simulink model "mainV02_49"  (R2016b)
settings: Solver=FixedStepAuto  StartTime=0.0  StopTime=inf  FixedStep=Ts  MaxStep=0.2  RelTol=1e-2
undefined symbols (not defined in the file): checks, datetime, decyear, deltae_degrees, deltafl_degrees, deltafr_degrees, deltar_degrees, deltat_1, deltat_2, deltat_3, deltat_4, deltat_5, Earth, F, ft, groundReaction, initialValues, juliandate, LD, leapyear, Light, m, MIL, Newton, Raphson, s, sigbuilder_block, Ts, Vehicle, WGS84
libraries: simulink x25, aerolibutil x17, aerolibtransform2 x12, aerolib6dofsys x5, aerolibasang x4, aerolib6dof2 x4, aerolibwind2 x3, aerolibbdyn x3, aerolibconvert2 x3, aerolibactuator x2, aerolibgravity2 x2, aerolibnav x2
(part 2 of 7)

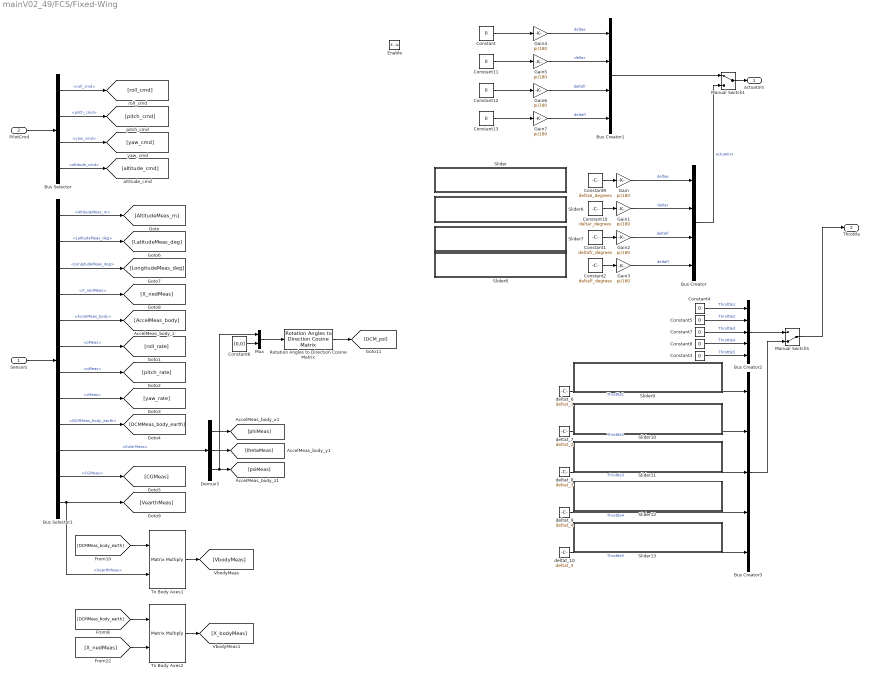
== system mainV02_49/FCS/Fixed-Wing ==
  Sensors : Inport  OutDataTypeStr=Bus: SensorsBus
  PilotCmd : Inport  Port=2  OutDataTypeStr=Bus: CommandBus
  Enable : EnablePort
  Bus Creator : BusCreator  Inputs='deltae','deltar','deltafr','deltafl'  OutDataTypeStr=Bus: ActuatorsBus  NonVirtualBus=on
  Bus Creator1 : BusCreator  Inputs='deltae','deltar','deltafr','deltafl'  OutDataTypeStr=Bus: ActuatorsBus  NonVirtualBus=on
  Bus Creator2 : BusCreator  Inputs='Throttle1','Throttle2','Throttle3','Throttle4','Throttle5'  OutDataTypeStr=Bus: ThrottleBus  NonVirtualBus=on
  Bus Creator3 : BusCreator  Inputs='Throttle1','Throttle2','Throttle3','Throttle4','Throttle5'  OutDataTypeStr=Bus: ThrottleBus  NonVirtualBus=on
  Bus Selector : BusSelector  OutputSignals=roll_cmd,pitch_cmd,yaw_cmd,altitude_cmd
  Bus Selector1 : BusSelector  OutputSignals=LLAMeas.AltitudeMeas_m,LLAMeas.LatitudeMeas_deg,LLAMeas.LongitudeMeas_deg,X_nedMeas,AccelMeas_body,OmegaMeas_body.pMeas,OmegaMeas_body.qMeas,OmegaMeas_body.rMeas,DCMMeas_body_earth,EulerMeas,CGMeas,VearthMeas
  Constant{,3..5,7..8,11..13} (9 alike) : Constant  Value=0
  Constant1 : Constant  Value=deltafr_degrees
  Constant10 : Constant  Value=deltar_degrees
  Constant2 : Constant  Value=deltafl_degrees
  Constant6 : Constant  Value=[0,0]
  Constant9 : Constant  Value=deltae_degrees
  Demux3 : Demux  Outputs=3
  Gain{,1..7} (8 alike) : Gain  Gain=pi/180
  Manual Switch1 : ManualSwitch
  Manual Switch5 : ManualSwitch  CurrentSetting=0
  Mux : Mux  Inputs=2
  Rotation Angles to Direction Cosine Matrix : aerolibtransform2/Rotation Angles to Direction Cosine Matrix  rotationOrder=ZYX
  Slider : Subsystem  DialogController=hmiCreateDDGDialog  IsWebBlock=on  mask(MWDashboardBlock){webBlockId=14b23d13-a400-494b-8ed9-02e5a1d75a92, webBlockType=slider, ShowInLibBrowser=on, ShowInitialText=on, HMISrcModelName=mainV02_49}
      mask prompts: webBlockId "WebBlock Id"; webBlockType "WebBlock Type"; HMISrcModelName "Source Model"
      mask help: SimulinkHMI:dialogs:SliderDialogDesc
      mask Help: helpview([docroot '/mapfiles/simulink.map'], 'hmi_slider')
      mask Display:
      | if strcmp(get_param(bdroot(gcb),'BlockDiagramType'), 'library')
      |     image([(matlabroot) '/toolbox/simulink/hmi/icons/Slider.png']);
      | end
  Slider10 : Subsystem  DialogController=hmiCreateDDGDialog  IsWebBlock=on  mask(MWDashboardBlock){webBlockId=64fa6611-4453-4c5a-8fed-f588a42e496e, webBlockType=slider, ShowInLibBrowser=on, ShowInitialText=on, HMISrcModelName=mainV02_49}
      mask prompts: webBlockId "WebBlock Id"; webBlockType "WebBlock Type"; HMISrcModelName "Source Model"
      mask help: SimulinkHMI:dialogs:SliderDialogDesc
      mask Help: helpview([docroot '/mapfiles/simulink.map'], 'hmi_slider')
      mask Display:
      | if strcmp(get_param(bdroot(gcb),'BlockDiagramType'), 'library')
      |     image([(matlabroot) '/toolbox/simulink/hmi/icons/Slider.png']);
      | end
  Slider11 : Subsystem  DialogController=hmiCreateDDGDialog  IsWebBlock=on  mask(MWDashboardBlock){webBlockId=9533f27f-d213-4a1e-af4f-df3e89cb42b9, webBlockType=slider, ShowInLibBrowser=on, ShowInitialText=on, HMISrcModelName=mainV02_49}
      mask prompts: webBlockId "WebBlock Id"; webBlockType "WebBlock Type"; HMISrcModelName "Source Model"
      mask help: SimulinkHMI:dialogs:SliderDialogDesc
      mask Help: helpview([docroot '/mapfiles/simulink.map'], 'hmi_slider')
      mask Display:
      | if strcmp(get_param(bdroot(gcb),'BlockDiagramType'), 'library')
      |     image([(matlabroot) '/toolbox/simulink/hmi/icons/Slider.png']);
      | end
  Slider12 : Subsystem  DialogController=hmiCreateDDGDialog  IsWebBlock=on  mask(MWDashboardBlock){webBlockId=b1a90b42-9e20-4e98-9400-f4073a2edd03, webBlockType=slider, ShowInLibBrowser=on, ShowInitialText=on, HMISrcModelName=mainV02_49}
      mask prompts: webBlockId "WebBlock Id"; webBlockType "WebBlock Type"; HMISrcModelName "Source Model"
      mask help: SimulinkHMI:dialogs:SliderDialogDesc
      mask Help: helpview([docroot '/mapfiles/simulink.map'], 'hmi_slider')
      mask Display:
      | if strcmp(get_param(bdroot(gcb),'BlockDiagramType'), 'library')
      |     image([(matlabroot) '/toolbox/simulink/hmi/icons/Slider.png']);
      | end
  Slider13 : Subsystem  DialogController=hmiCreateDDGDialog  IsWebBlock=on  mask(MWDashboardBlock){webBlockId=3f53d0a3-a536-4819-a79a-261ce29de858, webBlockType=slider, ShowInLibBrowser=on, ShowInitialText=on, HMISrcModelName=mainV02_49}
      mask prompts: webBlockId "WebBlock Id"; webBlockType "WebBlock Type"; HMISrcModelName "Source Model"
      mask help: SimulinkHMI:dialogs:SliderDialogDesc
      mask Help: helpview([docroot '/mapfiles/simulink.map'], 'hmi_slider')
      mask Display:
      | if strcmp(get_param(bdroot(gcb),'BlockDiagramType'), 'library')
      |     image([(matlabroot) '/toolbox/simulink/hmi/icons/Slider.png']);
      | end
  Slider6 : Subsystem  DialogController=hmiCreateDDGDialog  IsWebBlock=on  mask(MWDashboardBlock){webBlockId=0a8845a4-7a41-4249-8bd0-83b7bb709b45, webBlockType=slider, ShowInLibBrowser=on, ShowInitialText=on, HMISrcModelName=mainV02_49}
      mask prompts: webBlockId "WebBlock Id"; webBlockType "WebBlock Type"; HMISrcModelName "Source Model"
      mask help: SimulinkHMI:dialogs:SliderDialogDesc
      mask Help: helpview([docroot '/mapfiles/simulink.map'], 'hmi_slider')
      mask Display:
      | if strcmp(get_param(bdroot(gcb),'BlockDiagramType'), 'library')
      |     image([(matlabroot) '/toolbox/simulink/hmi/icons/Slider.png']);
      | end
  Slider7 : Subsystem  DialogController=hmiCreateDDGDialog  IsWebBlock=on  mask(MWDashboardBlock){webBlockId=5d3f7e6f-9551-44ea-8738-138cd7f6102a, webBlockType=slider, ShowInLibBrowser=on, ShowInitialText=on, HMISrcModelName=mainV02_49}
      mask prompts: webBlockId "WebBlock Id"; webBlockType "WebBlock Type"; HMISrcModelName "Source Model"
      mask help: SimulinkHMI:dialogs:SliderDialogDesc
      mask Help: helpview([docroot '/mapfiles/simulink.map'], 'hmi_slider')
      mask Display:
      | if strcmp(get_param(bdroot(gcb),'BlockDiagramType'), 'library')
      |     image([(matlabroot) '/toolbox/simulink/hmi/icons/Slider.png']);
      | end
  Slider8 : Subsystem  DialogController=hmiCreateDDGDialog  IsWebBlock=on  mask(MWDashboardBlock){webBlockId=c93866b8-d73b-474f-a677-46d479bf762f, webBlockType=slider, ShowInLibBrowser=on, ShowInitialText=on, HMISrcModelName=mainV02_49}
      mask prompts: webBlockId "WebBlock Id"; webBlockType "WebBlock Type"; HMISrcModelName "Source Model"
      mask help: SimulinkHMI:dialogs:SliderDialogDesc
      mask Help: helpview([docroot '/mapfiles/simulink.map'], 'hmi_slider')
      mask Display:
      | if strcmp(get_param(bdroot(gcb),'BlockDiagramType'), 'library')
      |     image([(matlabroot) '/toolbox/simulink/hmi/icons/Slider.png']);
      | end
  Slider9 : Subsystem  DialogController=hmiCreateDDGDialog  IsWebBlock=on  mask(MWDashboardBlock){webBlockId=8597f763-0fcc-4c4e-9d3c-a5079949b770, webBlockType=slider, ShowInLibBrowser=on, ShowInitialText=on, HMISrcModelName=mainV02_49}
      mask prompts: webBlockId "WebBlock Id"; webBlockType "WebBlock Type"; HMISrcModelName "Source Model"
      mask help: SimulinkHMI:dialogs:SliderDialogDesc
      mask Help: helpview([docroot '/mapfiles/simulink.map'], 'hmi_slider')
      mask Display:
      | if strcmp(get_param(bdroot(gcb),'BlockDiagramType'), 'library')
      |     image([(matlabroot) '/toolbox/simulink/hmi/icons/Slider.png']);
      | end
  To Body Axes1 : Product  Multiplication=Matrix(*)  SaturateOnIntegerOverflow=on  InputSameDT=on  OutDataTypeStr=Inherit: Same as first input
  To Body Axes2 : Product  Multiplication=Matrix(*)  SaturateOnIntegerOverflow=on  InputSameDT=on  OutDataTypeStr=Inherit: Same as first input
  deltat_10 : Constant  Value=deltat_5
  deltat_6 : Constant  Value=deltat_1
  deltat_7 : Constant  Value=deltat_2
  deltat_8 : Constant  Value=deltat_3
  deltat_9 : Constant  Value=deltat_4
  actuators : Outport
  Throttle : Outport  Port=2  OutDataTypeStr=Bus: ThrottleBus
  wires:
  PilotCmd/1 -> Bus Selector/1
  Sensors/1 -> Bus Selector1/1
  Bus Selector1/1 -> [AltitudeMeas_m]  "<AltitudeMeas_m>"
  Bus Selector/1 -> [roll_cmd]  "<roll_cmd>"
  Bus Selector/2 -> [pitch_cmd]  "<pitch_cmd>"
  Bus Selector/3 -> [yaw_cmd]  "<yaw_cmd>"
  Bus Selector/4 -> [altitude_cmd]  "<altitude_cmd>"
  Bus Selector1/6 -> [roll_rate]  "<pMeas>"
  Bus Selector1/7 -> [pitch_rate]  "<qMeas>"
  Bus Selector1/8 -> [yaw_rate]  "<rMeas>"
  Bus Selector1/9 -> [DCMMeas_body_earth]  "<DCMMeas_body_earth>"
  Demux3/1 -> [phiMeas]
  Demux3/2 -> [thetaMeas]
  Demux3/3 -> Mux/1, [psiMeas]
  Bus Selector1/11 -> [CGMeas]  "<CGMeas>"
  Bus Selector1/2 -> [LatitudeMeas_deg]  "<LatitudeMeas_deg>"
  Bus Selector1/3 -> [LongitudeMeas_deg]  "<LongitudeMeas_deg>"
  Bus Selector1/5 -> [AccelMeas_body]  "<AccelMeas_body>"
  Bus Selector1/4 -> [X_nedMeas]  "<X_nedMeas>"
  Bus Selector1/12 -> To Body Axes1/2, [VearthMeas]  "<VearthMeas>"
  [DCMMeas_body_earth] -> To Body Axes1/1
  To Body Axes1/1 -> [VbodyMeas]
  To Body Axes2/1 -> [X_bodyMeas]
  [DCMMeas_body_earth] -> To Body Axes2/1
  [X_nedMeas] -> To Body Axes2/2
  Bus Selector1/10 -> Demux3/1  "<EulerMeas>"
  Constant6/1 -> Mux/2
  Mux/1 -> Rotation Angles to Direction Cosine Matrix/1
  Rotation Angles to Direction Cosine Matrix/1 -> [DCM_psi]
  Bus Creator/1 -> Manual Switch1/2  "actuators"
  Gain1/1 -> Bus Creator/2  "deltar"
  Gain2/1 -> Bus Creator/3  "deltafr"
  Gain3/1 -> Bus Creator/4  "deltafl"
  Gain/1 -> Bus Creator/1  "deltae"
  Constant10/1 -> Gain1/1
  Constant1/1 -> Gain2/1
  Constant2/1 -> Gain3/1
  Constant9/1 -> Gain/1
  Constant4/1 -> Bus Creator2/1  "Throttle1"
  Constant7/1 -> Bus Creator2/3  "Throttle3"
  Constant5/1 -> Bus Creator2/2  "Throttle2"
  Constant8/1 -> Bus Creator2/4  "Throttle4"
  Constant3/1 -> Bus Creator2/5  "Throttle5"
  deltat_6/1 -> Bus Creator3/1  "Throttle1"
  deltat_8/1 -> Bus Creator3/3  "Throttle3"
  deltat_7/1 -> Bus Creator3/2  "Throttle2"
  deltat_9/1 -> Bus Creator3/4  "Throttle4"
  deltat_10/1 -> Bus Creator3/5  "Throttle5"
  Bus Creator2/1 -> Manual Switch5/1
  Bus Creator3/1 -> Manual Switch5/2
  Manual Switch5/1 -> Throttle/1
  Gain5/1 -> Bus Creator1/2  "deltar"
  Gain6/1 -> Bus Creator1/3  "deltafr"
  Gain7/1 -> Bus Creator1/4  "deltafl"
  Gain4/1 -> Bus Creator1/1  "deltae"
  Bus Creator1/1 -> Manual Switch1/1
  Manual Switch1/1 -> actuators/1
  Constant/1 -> Gain4/1
  Constant13/1 -> Gain7/1
  Constant12/1 -> Gain6/1
  Constant11/1 -> Gain5/1

== system mainV02_49/FCS/Fixed-Wing --> Quadcopter ==
  Enable : EnablePort
  Bus Creator : BusCreator  Inputs='deltae','deltar','deltafr','deltafl'  OutDataTypeStr=Bus: ActuatorsBus  NonVirtualBus=on
  Bus Creator1 : BusCreator  Inputs='Throttle1','Throttle2','Throttle3','Throttle4','Throttle5'  OutDataTypeStr=Bus: ThrottleBus  NonVirtualBus=on
  Constant{1..2,9..10} (4 alike) : Constant  Value=30
  Constant{20..24} (5 alike) : Constant
  Gain{,1..3} (4 alike) : Gain  Gain=pi/180
  IC{,1..4} (5 alike) : InitialCondition  Value=0
  Actuators : Outport  OutDataTypeStr=Bus: ActuatorsBus
  Throttle : Outport  Port=2  OutDataTypeStr=Bus: ThrottleBus
  wires:
  Bus Creator/1 -> Actuators/1  "Actuators"
  Gain1/1 -> Bus Creator/2  "deltar"
  Gain2/1 -> Bus Creator/3  "deltafr"
  Gain3/1 -> Bus Creator/4  "deltafl"
  Gain/1 -> Bus Creator/1  "deltae"
  Constant10/1 -> Gain1/1
  Constant1/1 -> Gain2/1
  Constant2/1 -> Gain3/1
  Constant9/1 -> Gain/1
  Bus Creator1/1 -> Throttle/1  "Throttle"
  Constant21/1 -> IC/1  "Throttle1"
  Constant23/1 -> IC2/1  "Throttle3"
  Constant22/1 -> IC1/1  "Throttle2"
  Constant24/1 -> IC3/1  "Throttle4"
  Constant20/1 -> IC4/1  "Throttle5"
  IC/1 -> Bus Creator1/1  "Throttle1"
  IC3/1 -> Bus Creator1/4  "Throttle4"
  IC4/1 -> Bus Creator1/5  "Throttle5"
  IC2/1 -> Bus Creator1/3  "Throttle3"
  IC1/1 -> Bus Creator1/2  "Throttle2"
